simulink model "chap9_6sim"  (Simulink 3.00)
settings: Solver=ode5  StartTime=0.0  StopTime=3  FixedStep=0.001  RelTol=1e-3
settings Model: LastModifiedBy=liu

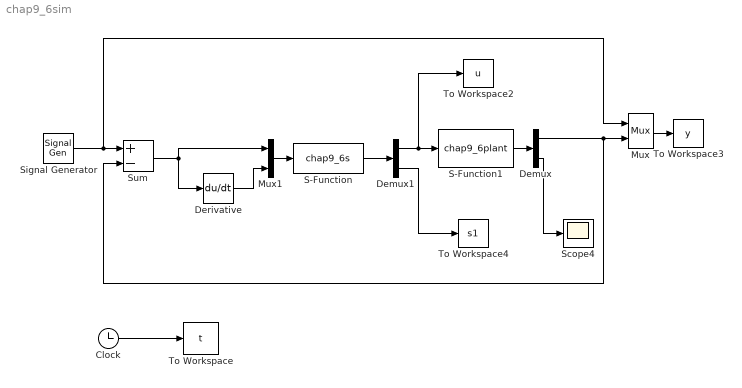
== system chap9_6sim ==
  Clock : Clock
      settings: DisplayTime=off  Decimation=10
  Demux : Demux  Outputs=2
  Demux1 : Demux  Outputs=2
  Derivative : Derivative
  Mux : Mux  Inputs=2
      settings: DisplayOption=none
  Mux1 : Mux  Inputs=2
  S-Function : S-Function  FunctionName=chap9_6s  PortCounts=[]  SFunctionModules=''
  S-Function1 : S-Function  FunctionName=chap9_6plant  PortCounts=[]  SFunctionModules=''
  Scope4 : Scope
      settings: TimeRange=3  YMin=-70  YMax=60  SaveToWorkspace=off  SaveName=ScopeData
  Signal Generator : SignalGenerator  WaveForm=sine  Amplitude=1  Frequency=3  Units=Hertz
  Sum : Sum  Inputs=+-  SaturateOnIntegerOverflow=on
  To Workspace : ToWorkspace  VariableName=t  SampleTime=-1  SaveFormat=Matrix
  To Workspace2 : ToWorkspace  VariableName=u  SampleTime=-1  SaveFormat=Matrix
  To Workspace3 : ToWorkspace  VariableName=y  SampleTime=-1  SaveFormat=Matrix
  To Workspace4 : ToWorkspace  VariableName=s1  SampleTime=-1  SaveFormat=Matrix
  wires:
  Signal Generator/1 -> Sum/1, Mux/1
  Mux1/1 -> S-Function/1
  Derivative/1 -> Mux1/2
  Sum/1 -> Derivative/1, Mux1/1
  S-Function/1 -> Demux1/1
  Clock/1 -> To Workspace/1
  Demux1/1 -> S-Function1/1, To Workspace2/1
  Demux1/2 -> To Workspace4/1
  S-Function1/1 -> Demux/1
  Mux/1 -> To Workspace3/1
  Demux/1 -> Mux/2, Sum/2
  Demux/2 -> Scope4/1
